simulink model "model"  (R2025a)
settings: Solver=VariableStepAuto  StartTime=0.0  StopTime=15  RelTol=1e-3
values from neighbouring files (symbols this model uses):
  K_d = 0.49    [setup.m]
  K_i = 4.9    [setup.m]
  K_p = 20    [setup.m]
settings Model: Creator=魏浩楠  LastModifiedBy=20174
settings RTWCC: GPUComputeCapability=3.5

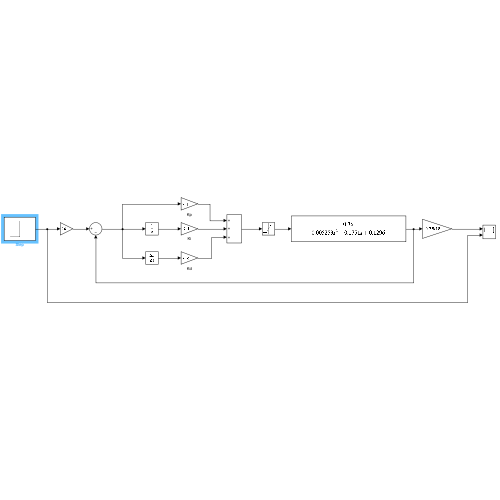
[thumbnail: Simulink's stored preview of the top-level diagram]
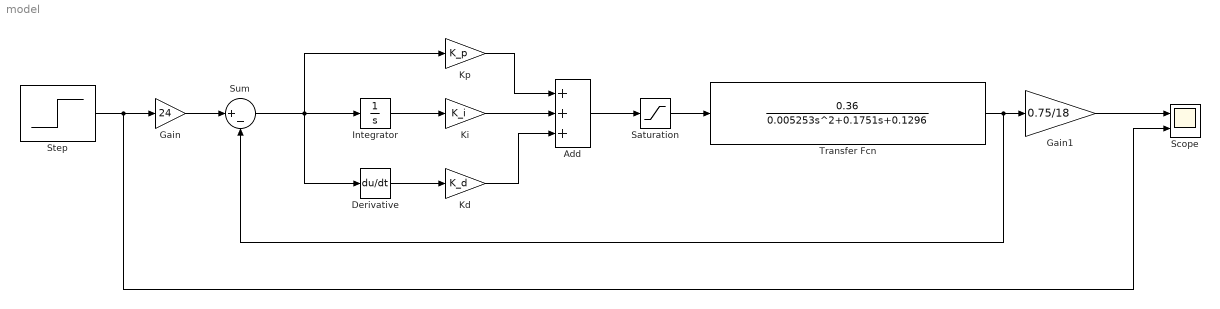
== system model ==
  Add : Sum  Inputs=+++
  Derivative : Derivative
  Gain : Gain  Gain=24
  Gain1 : Gain  Gain=0.75/18
  Integrator : Integrator
  Kd : Gain  Gain=K_d
  Ki : Gain  Gain=K_i
  Kp : Gain  Gain=K_p
  Saturation : Saturate  UpperLimit=1200  LowerLimit=-1200
  Scope : Scope  NumInputPorts=2
      settings: ActiveDisplayYMinimum=-0.43766552190797525  ActiveDisplayYMaximum=0.41454818036582919  YLabel=速度  DataLoggingVariableName=Data
  Step : Step  After=0.1  SampleTime=0
  Sum : Sum  Inputs=|+-
  Transfer Fcn : TransferFcn  Numerator=[0.36]  Denominator=[0.005253 0.1751 0.1296]
  wires:
  Step/1 -> Scope/2, Gain/1
  Gain/1 -> Sum/1
  Sum/1 -> Derivative/1, Kp/1, Integrator/1
  Integrator/1 -> Ki/1
  Derivative/1 -> Kd/1
  Kp/1 -> Add/1
  Ki/1 -> Add/2
  Kd/1 -> Add/3
  Add/1 -> Saturation/1
  Saturation/1 -> Transfer Fcn/1
  Transfer Fcn/1 -> Sum/2, Gain1/1
  Gain1/1 -> Scope/1
